simulink subsystem "LQI_classical"  (R2024a)
settings: Solver=VariableStepAuto  StartTime=0.0  StopTime=10.0  RelTol=1e-3
undefined symbols (not defined in the file): A, B, C, Continuous, D, K_LQI_classical, R, Time, u_eq, x_eq
libraries: ctrlSharedLib x1
settings Model: Creator=Bocchio  LastModifiedBy=Bocchio

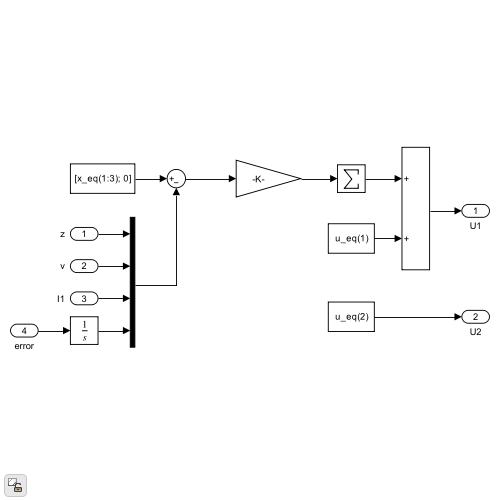
[thumbnail: Simulink's stored preview of the top-level diagram]
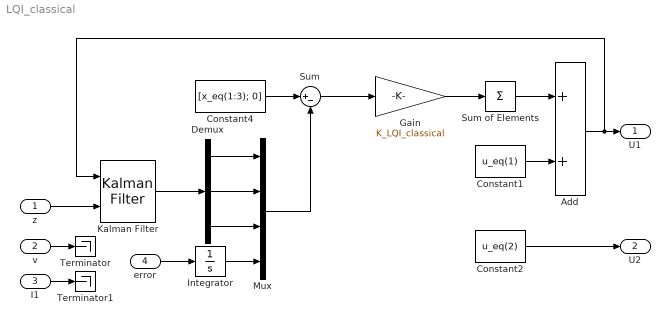
== system LQI_classical ==
  z : Inport
  v : Inport  Port=2
  I1 : Inport  Port=3
  error : Inport  Port=4
  Add : Sum
  Constant1 : Constant  Value=u_eq(1)
  Constant2 : Constant  Value=u_eq(2)
  Constant4 : Constant  Value=[x_eq(1:3); 0]
  Demux : Demux  Outputs=3
  Gain : Gain  Gain=K_LQI_classical
  Integrator : Integrator
  Kalman Filter : ctrlSharedLib/Kalman Filter  TimeDomain=Continuous-Time  UseCurrentEstimator=on  ModelSource=Individual A, B, C, D matrices  ModelSourceVariable=ss(0.95,1,1,0,1)  A=A  B=B  C=C  D=D  NumberOfStates=1  NumberOfInputs=1  NumberOfOutputs=1  InitialEstimateSource=Dialog  X0=0  P0=10  UseK=off  UseGH=off  NumberOfProcessNoiseInputs=1  G=1  TimeInvariantG=on  H=0  TimeInvariantH=on  Q=Q  TimeInvariantQ=on  R=R  TimeInvariantR=on  N=0  TimeInvariantN=on  AddInputPort=on  AddEnablePort=off  OutputEstimatedY=off  OutputP=off  Ts=-1
  Mux : Mux
  Sum : Sum  Inputs=|+-
  Sum of Elements : Sum  Inputs=+  CollapseDim=2
  Terminator : Terminator
  Terminator1 : Terminator
  U1 : Outport
  U2 : Outport  Port=2
  wires:
  error/1 -> Integrator/1
  Integrator/1 -> Mux/4
  Gain/1 -> Sum of Elements/1
  Demux/1 -> Mux/1
  Constant1/1 -> Add/2
  Sum/1 -> Gain/1
  Demux/3 -> Mux/3
  Sum of Elements/1 -> Add/1
  Constant4/1 -> Sum/1
  Constant2/1 -> U2/1
  Demux/2 -> Mux/2
  Add/1 -> U1/1, Kalman Filter/1
  Mux/1 -> Sum/2
  Kalman Filter/1 -> Demux/1
  z/1 -> Kalman Filter/2
  v/1 -> Terminator/1
  I1/1 -> Terminator1/1
